simulink model "MASH20_Bader_fixed_point2"  (R2024a)
settings: Solver=ode45  StartTime=0.0  StopTime=1  MaxStep=Ts/10  EnableMultiTasking=on
PreLoadFcn:
  | s0=sprintf('===========================================================================');disp(s0)
  | s1=sprintf('= Created by Bader Almutair bmutairi@kacst.edu.sa                         =');disp(s1)
  | s2=sprintf('= Date 12/11/2014                                                         =');disp(s2)
  | s3=sprintf('= Refer to the PhD thesis Ch4,P.55                                        =');disp(s3)
  | s4=sprintf('===========================================================================');disp(s4)
values from neighbouring files (symbols this model uses):
  AA = AA_design*(mismatch_lower_limit + rand_range*rand)    [simon_test.m]    (also in testPSD_simulink.m)
  acceleration_enable = 1    [simon_test.m]    (also in testPSD_simulink.m)
  b = b_design*(0.8 + (1.2 - 0.8) * rand)    [D2_parameter_mapping.m]    (also in simon_test.m = b_design*(mismatch_lower_limit + rand_range*rand); testPSD_simulink.m = b_design*(mismatch_lower_limit + rand_range*rand))
  clk = i    [GA_multipleruns_TB.m]    (also in GA_multipleruns_TB_c2d.m)
  d0 = d0_design*(mismatch_lower_limit + rand_range*rand)    [simon_test.m]    (also in testPSD_simulink.m)
  electronic_noise_enable = 1    [simon_test.m]    (also in testPSD_simulink.m)
  enoise = 10e-9    (= 1e-08)    [simon_test.m]    (also in testPSD_simulink.m)
  epsilon = 8.854e-12    [population_score_c2d.m]    (also in simon_test.m; testPSD_c2d.m; testPSD_simulink.m)
  Finput = F_resolution*128    (= 260.4140625)    [new_generation_coeff.m]    (also in simon_test.m; testPSD_simulink.m)
  k = k_design*(0.8 + (1.2 - 0.8) * rand)    [D2_parameter_mapping.m]    (also in log2_linear_taylor.m = floor(log2(x)); population_score.m = floor(log2(real(Y3).^2 + imag(Y3).^2)); population_score_c2d.m = floor(log2(Y3)); simon_test.m = k_design*(mismatch_lower_limit + rand_range*rand))
  Kfb = Kfb_design*(0.8 + (1.2 - 0.8) * rand)    [D2_parameter_mapping.m]    (also in simon_test.m = 0.5*epsilon*AA*(Vfeedback^2)/(d0^2); testPSD_simulink.m = 0.5*epsilon*AA*(Vfeedback^2)/(d0^2))
  Kpo = Kpo_design*(0.8 + (1.2 - 0.8) * rand)    [D2_parameter_mapping.m]    (also in simon_test.m = Kpo_design*(mismatch_lower_limit + rand_range*rand); testPSD_simulink.m = Kpo_design*(mismatch_lower_limit + rand_range*rand))
  Lfactor = Vfeedback/d0    [simon_test.m]    (also in testPSD_simulink.m)
  m = m_design*(0.8 + (1.2 - 0.8) * rand)    [D2_parameter_mapping.m]    (also in simon_test.m = m_design*(mismatch_lower_limit + rand_range*rand); testPSD_simulink.m = m_design*(mismatch_lower_limit + rand_range*rand))
  Ts = 1/Fs    (= 7.50007500075e-06)    [new_generation_coeff.m]    (also in simon_test.m; simple_fft_test.m = 1/F; testPSD_c2d.m; testPSD_simulink.m)
  Vfeedback = Vfeedback_design*(mismatch_lower_limit + rand_range*rand)    [simon_test.m]    (also in testPSD_simulink.m)
  x = linspace(min(a4), max(a4), 100)    [D2_parameter_mapping.m]    (also in log2_linear_taylor.m = 1e-10; simon_test.m = 0.9; testPSD_simulink.m = 0.9)
undefined symbols (not defined in the file or in its folder): clk_enable, D2den, reset_x
libraries: hdlmdlgenlib x4, simulink x3, simulink_extras x2, dspsigops x1, vivadosimlib x1
settings Model: Creator=Administrator  LastModifiedBy=Simon
settings SolverCC: AlgebraicLoopSolver=TrustRegion
settings DataIOCC: LimitDataPoints=on  SaveFormat=Array  SignalLoggingSaveFormat=ModelDataLogs  ReturnWorkspaceOutputs=off
settings OptimizationCC: ReuseModelBlockBuffer=off  ExpressionDepthLimit=2147483647  LifeSpan=inf
settings DebuggingCC: UnderspecifiedInitializationDetection=Classic  MergeDetectMultiDrivingBlocksExec=none  SolverPrmCheckMsg=warning  FcnCallInpInsideContextMsg=warning  UnconnectedInputMsg=warning  UnconnectedOutputMsg=warning  UnconnectedLineMsg=warning  StateNameClashWarn=warning  SFUnexpectedBacktrackingDiag=warning  SFNoUnconditionalDefaultTransitionDiag=warning  SFExecutionAtInitializationDiag=none  ArithmeticOperatorsInVariantConditions=warning
settings HardwareCC: ProdBitPerPointer=32  ProdBitPerSizeT=32  ProdBitPerPtrDiffT=32  ProdLargestAtomicFloat=None  ProdIntDivRoundTo=Undefined  ProdEndianess=Unspecified  ProdWordSize=32  ProdHWDeviceType=32-bit Generic
settings ModelReferenceCC: PropagateSignalLabelsOutOfModel=off
settings SFSimCC: SimUseLocalCustomCode=off  CustomCodeUndefinedFunction=UseInterfaceOnly
settings RTWCC: RTWUseLocalCustomCode=off  GPUComputeCapability=3.5
settings CodeAppCC: StateflowObjectComments=on
settings GRTTargetCC: TargetLangStandard=C89/C90 (ANSI)  CombineOutputUpdateFcns=off  GRTInterface=on
settings ConfigComp: CovMetricSettings=dw  CovSaveCumulativeToWorkspaceVar=on  CovSaveSingleToWorkspaceVar=on  CovExternalEMLEnable=off

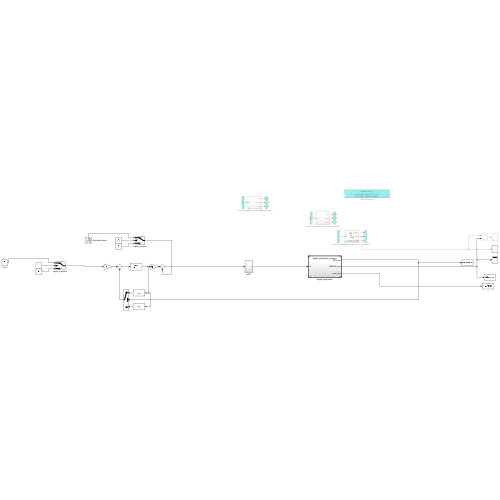
[thumbnail: Simulink's stored preview of the top-level diagram]
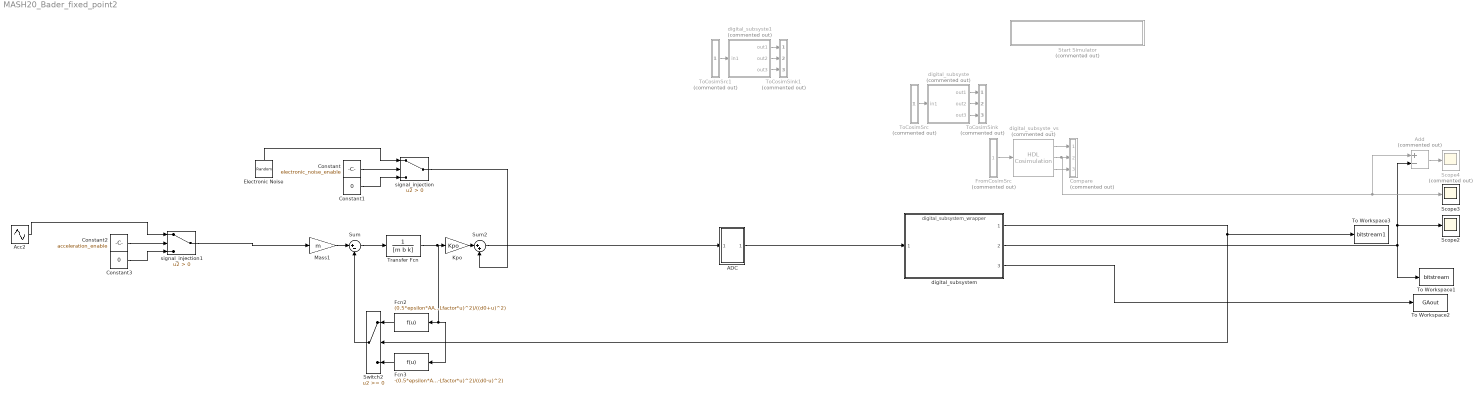
== system MASH20_Bader_fixed_point2 ==
  ADC : Subsystem
  Acc2 : Sin  Amplitude=(Kfb/m)*x  Frequency=Finput*2*pi  SampleTime=0
  Add : Sum  Commented=on  Inputs=+-
  Compare : Subsystem  Commented=on
      mask Display: disp('')
  Constant : Constant  Value=electronic_noise_enable  OutDataTypeStr=boolean  SampleTime=Ts
  Constant1 : Constant  Value=0  OutDataTypeStr=boolean  SampleTime=Ts
  Constant2 : Constant  Value=acceleration_enable  OutDataTypeStr=boolean  SampleTime=Ts
  Constant3 : Constant  Value=0  OutDataTypeStr=boolean  SampleTime=Ts
  Electronic Noise : RandomNumber  Variance=(enoise*sqrt(5/Ts))^2  Seed=432  SampleTime=Ts
  Fcn2 : Fcn  Expr=(0.5*epsilon*AA*(Vfeedback+Lfactor*u)^2)/((d0+u)^2)
  Fcn3 : Fcn  Expr=-(0.5*epsilon*AA*(Vfeedback-Lfactor*u)^2)/((d0-u)^2)
  FromCosimSrc : Subsystem  Commented=on
      mask Display: disp('')
  Kpo : Gain  Gain=Kpo
  Mass1 : Gain  Gain=m
  Scope2 : Scope
  Scope3 : Scope
  Scope4 : Scope  Commented=on
  Start Simulator : Subsystem  Commented=on
      settings: OpenFcn=|
      | cosimDirName = pwd;
      | cd 'hdl_prj_xd\hdlsrc\digital_subsystem_wrapper';
      | [s,r] = system('vivado -mode batch -source gm_digital_subsystem_wrapper_vs.tcl','-echo');
      | cd (cosimDirName);
      | clear cosimDirName;
      | if s
      |    error('Failed to create Vivado HDL design DLL using script gm_digital_subsystem_wrapper_vs.tcl.');
      | end
      mask Display: disp('Double-click to\nregenerate Vivado HDL DLL\nfor design digital_subsyste')
  Sum : Sum  Inputs=|+-
  Sum2 : Sum  Inputs=|++
  Switch2 : Switch  SaturateOnIntegerOverflow=off  InputSameDT=off
  To Workspace1 : ToWorkspace  VariableName=bitstream  SampleTime=Ts
  To Workspace2 : ToWorkspace  VariableName=GAout  SampleTime=Ts
  To Workspace3 : ToWorkspace  VariableName=bitstream1  SampleTime=Ts
  ToCosimSink : Subsystem  Commented=on
      mask Display: disp('')
  ToCosimSink1 : Subsystem  Commented=on
      mask Display: disp('')
  ToCosimSrc : Subsystem  Commented=on
      mask Display: disp('')
  ToCosimSrc1 : Subsystem  Commented=on
      mask Display: disp('')
  Transfer Fcn : TransferFcn  Denominator=[m b k]
  digital_subsyste : Subsystem  Commented=on
  digital_subsyste1 : Subsystem  Commented=on
  digital_subsyste_vs : vivadosimlib/HDL Cosimulation  Commented=on  PortPaths=/digital_subsyste/in1;/digital_subsyste/out1;/digital_subsyste/out2;/digital_subsyste/out3  PortModes=[1 2 2 2 ]  PortTimes=[-1 7.5000750007500073716719922456430680313133052550256252288818359375e-06 7.5000750007500073716719922456430680313133052550256252288818359375e-06 7.5000750007500073716719922456430680313133052550256252288818359375e-06 ]  PortSigns=[-1 1 1 1 ]  PortFracLengths=[0,32,32,32]  PortWordLengths=[-1,64,64,64]  PortHDLWordSizes=[64,64,64,64]  CommLocal=on  CommSharedMemory=on  CommPortNumber=4449  CommShowInfo=on  ClockPaths=clk;clk_enable;reset_x;  ClockModes=[2 4 4]  ClockTimes=[1e-08 3.7e-08 2.7e-08]  TclPreSimCommand="puts \"Running Simulink Cosimulation block.\""  TclPostSimCommand="puts \"done\""  TimingMode=ns  TimingScaleFactor=1333320  idxCellArray={'UNUSED_VAR'}  CosimBypass=Full Simulation  AllowDirectFeedthrough=on  ProductName=EDA Simulator Link VS  RunAutoTimescale=off  HdlClocks=0  PreRunTime=40  PreRunTimeUnit=ns
  digital_subsystem : ModelReference  ModelNameDialog=digital_subsystem_wrapper  SimulationMode=Normal  ModelReferenceVersion=24.17
  signal_injection : Switch  Criteria=u2 > Threshold  SaturateOnIntegerOverflow=off  InputSameDT=off  OutDataTypeStr=Inherit: Same as first input
  signal_injection1 : Switch  Criteria=u2 > Threshold  SaturateOnIntegerOverflow=off  InputSameDT=off  OutDataTypeStr=Inherit: Same as first input
  wires:
  Transfer Fcn/1 -> Fcn3/1, Fcn2/1, Kpo/1
  Sum/1 -> Transfer Fcn/1
  Mass1/1 -> Sum/1
  Fcn2/1 -> Switch2/1
  Fcn3/1 -> Switch2/3
  Switch2/1 -> Sum/2
  Kpo/1 -> Sum2/1
  digital_subsystem/1 -> Switch2/2, To Workspace3/1
  digital_subsystem/2 -> To Workspace1/1, Add/2, Scope2/1
  digital_subsystem/3 -> To Workspace2/1
  digital_subsyste_vs/2 -> Add/1, Scope3/1, Compare/2(in2)
  FromCosimSrc/1(out1) -> digital_subsyste_vs/1
  digital_subsyste_vs/3 -> Compare/3(in3)
  digital_subsyste_vs/1 -> Compare/1(in1)
  Add/1 -> Scope4/1
  Sum2/1 -> ADC/1(In1)
  digital_subsyste/2(out2) -> ToCosimSink/2(in2)
  digital_subsyste/1(out1) -> ToCosimSink/1(in1)
  ToCosimSrc/1(out1) -> digital_subsyste/1(in1)
  digital_subsyste/3(out3) -> ToCosimSink/3(in3)
  ADC/1(Out1) -> digital_subsystem/1
  ToCosimSrc1/1(out1) -> digital_subsyste1/1(in1)
  digital_subsyste1/1(out1) -> ToCosimSink1/1(in1)
  digital_subsyste1/3(out3) -> ToCosimSink1/3(in3)
  digital_subsyste1/2(out2) -> ToCosimSink1/2(in2)
  Constant1/1 -> signal_injection/3
  Electronic Noise/1 -> signal_injection/1
  Constant/1 -> signal_injection/2
  signal_injection/1 -> Sum2/2
  Constant2/1 -> signal_injection1/2
  Acc2/1 -> signal_injection1/1
  Constant3/1 -> signal_injection1/3
  signal_injection1/1 -> Mass1/1

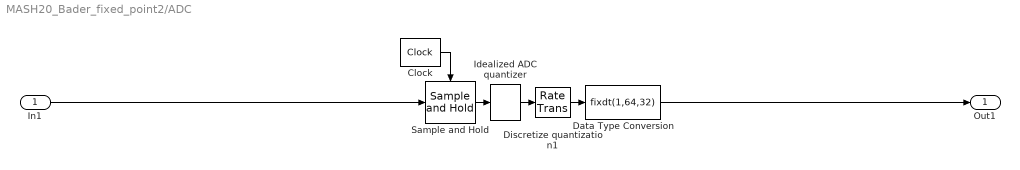
== system MASH20_Bader_fixed_point2/ADC ==
  In1 : Inport
  Clock : simulink_extras/Flip Flops/Clock  period=Ts
  Data Type Conversion : DataTypeConversion  OutDataTypeStr=fixdt(1,64,32)  SaturateOnIntegerOverflow=off  RndMeth=Floor
  Discretize quantization1 : RateTransition  OutPortSampleTime=Ts
  Idealized ADC quantizer : simulink_extras/Additional Discrete/Idealized ADC quantizer  NumberOfConverterBits=12  Vmin=-2.5  Vmax=2.5  OutputDataType=double  OutputNegativeValues=on
  Sample and Hold : dspsigops/Sample and Hold  trig=Rising edge  initCond=0  latchinput=off
  Out1 : Outport
  wires:
  Discretize quantization1/1 -> Data Type Conversion/1
  Idealized ADC quantizer/1 -> Discretize quantization1/1
  Clock/1 -> Sample and Hold/Trigger
  In1/1 -> Sample and Hold/1
  Data Type Conversion/1 -> Out1/1
  Sample and Hold/1 -> Idealized ADC quantizer/1

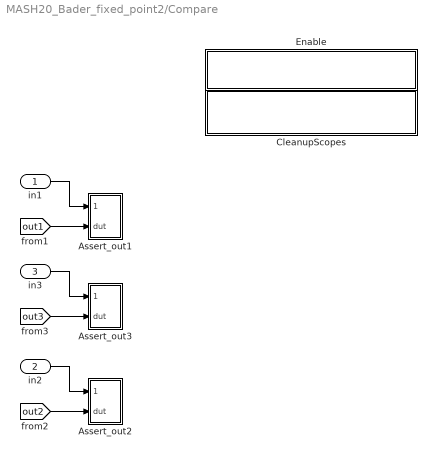
== system MASH20_Bader_fixed_point2/Compare ==
  in1 : Inport
  in2 : Inport  Port=2
  in3 : Inport  Port=3
  Assert_out1 : Subsystem
      settings: LibrarySourceBlock=hdlmdlgenlib/AssertEq
  Assert_out2 : Subsystem
      settings: LibrarySourceBlock=hdlmdlgenlib/AssertEq
  Assert_out3 : Subsystem
      settings: LibrarySourceBlock=hdlmdlgenlib/AssertEq
  CleanupScopes : Subsystem
      settings: OpenFcn=|
      | blkName = gcb; %self block
      | idx = regexp(blkName, '/CleanupScopes$', 'once');
      | blkParent = blkName(1:idx-1);
      | blks=find_system(blkParent, 'LookUnderMasks', 'all','blocktype', 'Scope');
      | for itr = 1:length(blks)
      | 	 hScopeCfg = get_param(blks{itr},'ScopeConfiguration');
      | 	 hScopeCfg.Visible = ~ hScopeCfg.Visible;
      | end
      | drawnow;
      mask Display: fprintf(message('hdlcoder:cosim:vnl_dblclick').getString());
  Enable : Subsystem
      settings: OpenFcn=|
      | blkName = gcb;
      | idx = regexp(blkName, '/Enable$', 'once');
      | blkParent = blkName(1:idx-1);
      | blks=find_system(blkParent, 'LookUnderMasks', 'all','blocktype', 'Assertion');
      | e = get_param(blks{1}, 'Enabled');
      | if strcmp(e, 'on'), f= 'off';, else, f = 'on';, end
      | for ii=1:length(blks), set_param(blks{ii}, 'Enabled', f);, end
      | set_param(gcb, 'MaskDisplay',['fprintf(message(''hdlcoder:cosim:vnl_dblclick_assertions'',','''',upper(e),'''',').getString())']);
      mask Display: fprintf(message('hdlcoder:cosim:vnl_dblclick_assertions','OFF').getString());
  wires:
  [out3] -> Assert_out3/2(dut)
  in3/1 -> Assert_out3/1(cosim)
  in1/1 -> Assert_out1/1(cosim)
  in2/1 -> Assert_out2/1(cosim)
  [out1] -> Assert_out1/2(dut)
  [out2] -> Assert_out2/2(dut)

== system MASH20_Bader_fixed_point2/FromCosimSrc ==
  out1 : Outport
  wires:
  [in1] -> out1/1

== system MASH20_Bader_fixed_point2/Start Simulator ==

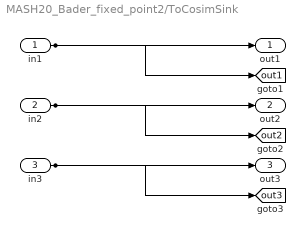
== system MASH20_Bader_fixed_point2/ToCosimSink ==
  in1 : Inport
  in2 : Inport  Port=2
  in3 : Inport  Port=3
  out1 : Outport
  out2 : Outport  Port=2
  out3 : Outport  Port=3
  tag scope: out1=global, out2=global, out3=global
  wires:
  in1/1 -> out1/1, [out1]
  in2/1 -> out2/1, [out2]
  in3/1 -> out3/1, [out3]

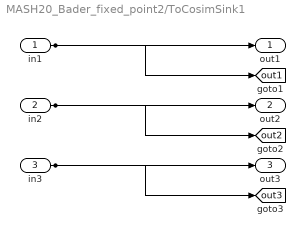
== system MASH20_Bader_fixed_point2/ToCosimSink1 ==
  in1 : Inport
  in2 : Inport  Port=2
  in3 : Inport  Port=3
  out1 : Outport
  out2 : Outport  Port=2
  out3 : Outport  Port=3
  tag scope: out1=global, out2=global, out3=global
  wires:
  in1/1 -> out1/1, [out1]
  in2/1 -> out2/1, [out2]
  in3/1 -> out3/1, [out3]

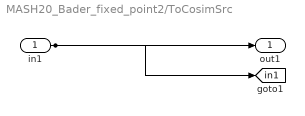
== system MASH20_Bader_fixed_point2/ToCosimSrc ==
  in1 : Inport
  out1 : Outport
  tag scope: in1=global
  wires:
  in1/1 -> out1/1, [in1]

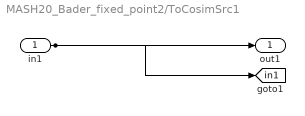
== system MASH20_Bader_fixed_point2/ToCosimSrc1 ==
  in1 : Inport
  out1 : Outport
  tag scope: in1=global
  wires:
  in1/1 -> out1/1, [in1]

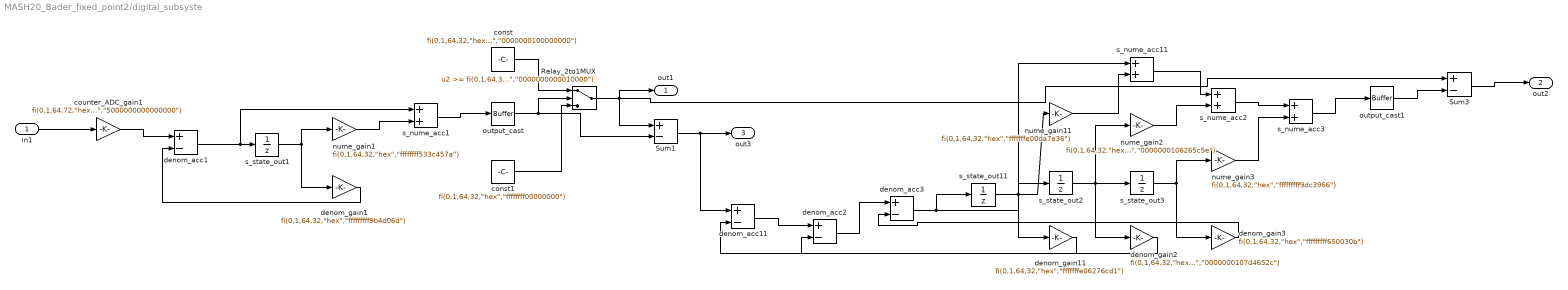
== system MASH20_Bader_fixed_point2/digital_subsyste ==
  in1 : Inport  OutDataTypeStr=fixdt(1, 64, 32)  PortDimensions=1  SampleTime=7.50007500075001e-06
  Relay_2to1MUX : Switch  Threshold="fi(0,1,64,32,\"hex\",\"0000000000010000\")"  OutDataTypeStr=fixdt(1, 64, 32)  SampleTime=7.50007500075001e-06  SaturateOnIntegerOverflow=off  InputSameDT=off
  Sum1 : Sum  Inputs=+-  OutDataTypeStr=fixdt(1, 64, 32)  AccumDataTypeStr=fixdt(1, 64, 32)  SampleTime=7.50007500075001e-06
  Sum3 : Sum  Inputs=+-  OutDataTypeStr=fixdt(1, 64, 32)  AccumDataTypeStr=fixdt(1, 64, 32)  SampleTime=7.50007500075001e-06
  const : Constant  Value="fi(0,1,64,32,\"hex\",\"0000000100000000\")"  OutDataTypeStr=fixdt(1, 64, 32)  SampleTime=7.50007500075001e-06
  const1 : Constant  Value="fi(0,1,64,32,\"hex\",\"ffffffff00000000\")"  OutDataTypeStr=fixdt(1, 64, 32)  SampleTime=7.50007500075001e-06
  counter_ADC_gain1 : Gain  Gain="fi(0,1,64,72,\"hex\",\"5000000000000000\")"  ParamDataTypeStr=fixdt(1, 64, 72)  OutDataTypeStr=fixdt(1, 64, 32)  SampleTime=7.50007500075001e-06
  denom_acc{1..3,11} (4 alike) : Sum  Inputs=+-  OutDataTypeStr=fixdt(1, 64, 32)  AccumDataTypeStr=fixdt(1, 64, 32)  SampleTime=7.50007500075001e-06
  denom_gain1 : Gain  Gain="fi(0,1,64,32,\"hex\",\"fffffffff9b4d06d\")"  ParamDataTypeStr=fixdt(1, 64, 32)  OutDataTypeStr=fixdt(1, 64, 32)  SampleTime=7.50007500075001e-06
  denom_gain11 : Gain  Gain="fi(0,1,64,32,\"hex\",\"fffffffe06276cd1\")"  ParamDataTypeStr=fixdt(1, 64, 32)  OutDataTypeStr=fixdt(1, 64, 32)  SampleTime=7.50007500075001e-06
  denom_gain2 : Gain  Gain="fi(0,1,64,32,\"hex\",\"0000000107d4652c\")"  ParamDataTypeStr=fixdt(1, 64, 32)  OutDataTypeStr=fixdt(1, 64, 32)  SampleTime=7.50007500075001e-06
  denom_gain3 : Gain  Gain="fi(0,1,64,32,\"hex\",\"fffffffff650030b\")"  ParamDataTypeStr=fixdt(1, 64, 32)  OutDataTypeStr=fixdt(1, 64, 32)  SampleTime=7.50007500075001e-06
  nume_gain1 : Gain  Gain="fi(0,1,64,32,\"hex\",\"ffffffff533c457a\")"  ParamDataTypeStr=fixdt(1, 64, 32)  OutDataTypeStr=fixdt(1, 64, 32)  SampleTime=7.50007500075001e-06
  nume_gain11 : Gain  Gain="fi(0,1,64,32,\"hex\",\"fffffffe00da7e36\")"  ParamDataTypeStr=fixdt(1, 64, 32)  OutDataTypeStr=fixdt(1, 64, 32)  SampleTime=7.50007500075001e-06
  nume_gain2 : Gain  Gain="fi(0,1,64,32,\"hex\",\"0000000106265c5e\")"  ParamDataTypeStr=fixdt(1, 64, 32)  OutDataTypeStr=fixdt(1, 64, 32)  SampleTime=7.50007500075001e-06
  nume_gain3 : Gain  Gain="fi(0,1,64,32,\"hex\",\"fffffffff9dc3966\")"  ParamDataTypeStr=fixdt(1, 64, 32)  OutDataTypeStr=fixdt(1, 64, 32)  SampleTime=7.50007500075001e-06
  output_cast : hdlmdlgenlib/Buffer
  output_cast1 : hdlmdlgenlib/Buffer
  s_nume_acc{1..3,11} (4 alike) : Sum  OutDataTypeStr=fixdt(1, 64, 32)  SampleTime=7.50007500075001e-06
  s_state_out{1..3,11} (4 alike) : UnitDelay  InitialCondition="fi(0,1,64,32,\"hex\",\"0000000000000000\")"  SampleTime=7.50007500075001e-06
  out1 : Outport  SampleTime=7.50007500075001e-06
  out2 : Outport  Port=2  SampleTime=7.50007500075001e-06
  out3 : Outport  Port=3  SampleTime=7.50007500075001e-06
  wires:
  const1/1 -> Relay_2to1MUX/3
  const/1 -> Relay_2to1MUX/1
  output_cast1/1 -> Sum3/2
  s_nume_acc3/1 -> output_cast1/1
  s_nume_acc2/1 -> s_nume_acc3/1
  s_nume_acc11/1 -> s_nume_acc2/1
  nume_gain3/1 -> s_nume_acc3/2
  nume_gain2/1 -> s_nume_acc2/2
  nume_gain11/1 -> s_nume_acc11/2
  denom_gain3/1 -> denom_acc3/2
  denom_gain2/1 -> denom_acc2/2
  denom_gain11/1 -> denom_acc11/2
  s_state_out3/1 -> denom_gain3/1, nume_gain3/1
  s_state_out2/1 -> s_state_out3/1, denom_gain2/1, nume_gain2/1
  s_state_out11/1 -> s_state_out2/1, denom_gain11/1, nume_gain11/1
  denom_acc3/1 -> s_nume_acc11/1, s_state_out11/1
  denom_acc2/1 -> denom_acc3/1
  denom_acc11/1 -> denom_acc2/1
  output_cast/1 -> Relay_2to1MUX/2, Sum1/2
  s_nume_acc1/1 -> output_cast/1
  nume_gain1/1 -> s_nume_acc1/2
  denom_gain1/1 -> denom_acc1/2
  s_state_out1/1 -> denom_gain1/1, nume_gain1/1
  denom_acc1/1 -> s_nume_acc1/1, s_state_out1/1
  counter_ADC_gain1/1 -> denom_acc1/1
  Sum3/1 -> out2/1
  Sum1/1 -> denom_acc11/1, out3/1
  Relay_2to1MUX/1 -> out1/1, Sum1/1, Sum3/1
  in1/1 -> counter_ADC_gain1/1

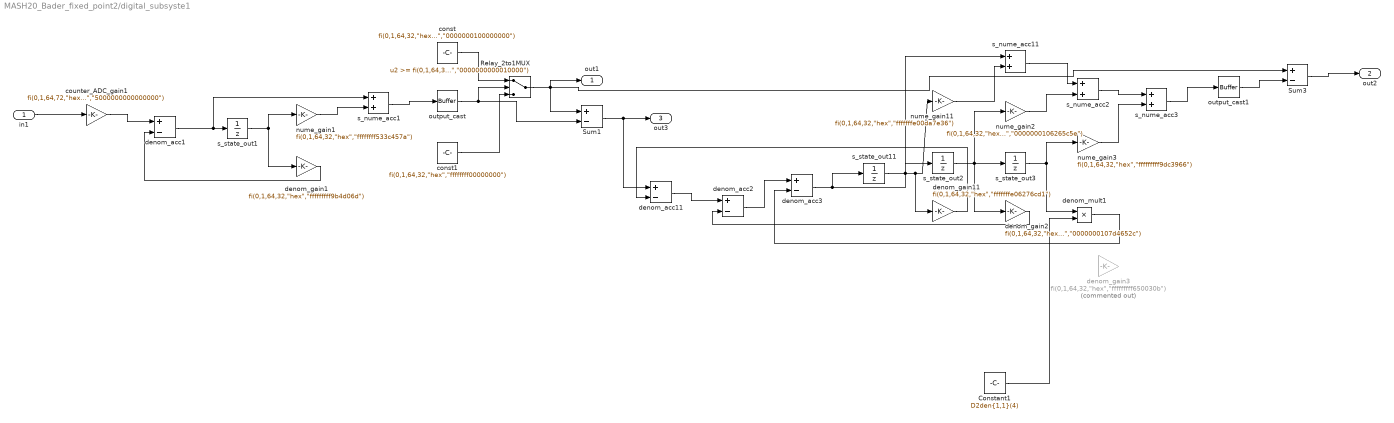
== system MASH20_Bader_fixed_point2/digital_subsyste1 ==
  in1 : Inport  OutDataTypeStr=fixdt(1, 64, 32)  PortDimensions=1  SampleTime=7.50007500075001e-06
  Constant1 : Constant  Value=D2den{1,1}(4)  OutDataTypeStr=fixdt(1,64,32)  SampleTime=Ts
  Relay_2to1MUX : Switch  Threshold="fi(0,1,64,32,\"hex\",\"0000000000010000\")"  OutDataTypeStr=fixdt(1, 64, 32)  SampleTime=7.50007500075001e-06  SaturateOnIntegerOverflow=off  InputSameDT=off
  Sum1 : Sum  Inputs=+-  OutDataTypeStr=fixdt(1, 64, 32)  AccumDataTypeStr=fixdt(1, 64, 32)  SampleTime=7.50007500075001e-06
  Sum3 : Sum  Inputs=+-  OutDataTypeStr=fixdt(1, 64, 32)  AccumDataTypeStr=fixdt(1, 64, 32)  SampleTime=7.50007500075001e-06
  const : Constant  Value="fi(0,1,64,32,\"hex\",\"0000000100000000\")"  OutDataTypeStr=fixdt(1, 64, 32)  SampleTime=7.50007500075001e-06
  const1 : Constant  Value="fi(0,1,64,32,\"hex\",\"ffffffff00000000\")"  OutDataTypeStr=fixdt(1, 64, 32)  SampleTime=7.50007500075001e-06
  counter_ADC_gain1 : Gain  Gain="fi(0,1,64,72,\"hex\",\"5000000000000000\")"  ParamDataTypeStr=fixdt(1, 64, 72)  OutDataTypeStr=fixdt(1, 64, 32)  SampleTime=7.50007500075001e-06
  denom_acc{1..3,11} (4 alike) : Sum  Inputs=+-  OutDataTypeStr=fixdt(1, 64, 32)  AccumDataTypeStr=fixdt(1, 64, 32)  SampleTime=7.50007500075001e-06
  denom_gain1 : Gain  Gain="fi(0,1,64,32,\"hex\",\"fffffffff9b4d06d\")"  ParamDataTypeStr=fixdt(1, 64, 32)  OutDataTypeStr=fixdt(1, 64, 32)  SampleTime=7.50007500075001e-06
  denom_gain11 : Gain  Gain="fi(0,1,64,32,\"hex\",\"fffffffe06276cd1\")"  ParamDataTypeStr=fixdt(1, 64, 32)  OutDataTypeStr=fixdt(1, 64, 32)  SampleTime=7.50007500075001e-06
  denom_gain2 : Gain  Gain="fi(0,1,64,32,\"hex\",\"0000000107d4652c\")"  ParamDataTypeStr=fixdt(1, 64, 32)  OutDataTypeStr=fixdt(1, 64, 32)  SampleTime=7.50007500075001e-06
  denom_gain3 : Gain  Commented=on  Gain="fi(0,1,64,32,\"hex\",\"fffffffff650030b\")"  ParamDataTypeStr=fixdt(1, 64, 32)  OutDataTypeStr=fixdt(1, 64, 32)  SampleTime=7.50007500075001e-06
  denom_mult1 : Product  OutDataTypeStr=fixdt(1,64,32)
  nume_gain1 : Gain  Gain="fi(0,1,64,32,\"hex\",\"ffffffff533c457a\")"  ParamDataTypeStr=fixdt(1, 64, 32)  OutDataTypeStr=fixdt(1, 64, 32)  SampleTime=7.50007500075001e-06
  nume_gain11 : Gain  Gain="fi(0,1,64,32,\"hex\",\"fffffffe00da7e36\")"  ParamDataTypeStr=fixdt(1, 64, 32)  OutDataTypeStr=fixdt(1, 64, 32)  SampleTime=7.50007500075001e-06
  nume_gain2 : Gain  Gain="fi(0,1,64,32,\"hex\",\"0000000106265c5e\")"  ParamDataTypeStr=fixdt(1, 64, 32)  OutDataTypeStr=fixdt(1, 64, 32)  SampleTime=7.50007500075001e-06
  nume_gain3 : Gain  Gain="fi(0,1,64,32,\"hex\",\"fffffffff9dc3966\")"  ParamDataTypeStr=fixdt(1, 64, 32)  OutDataTypeStr=fixdt(1, 64, 32)  SampleTime=7.50007500075001e-06
  output_cast : hdlmdlgenlib/Buffer
  output_cast1 : hdlmdlgenlib/Buffer
  s_nume_acc{1..3,11} (4 alike) : Sum  OutDataTypeStr=fixdt(1, 64, 32)  SampleTime=7.50007500075001e-06
  s_state_out{1..3,11} (4 alike) : UnitDelay  InitialCondition="fi(0,1,64,32,\"hex\",\"0000000000000000\")"  SampleTime=7.50007500075001e-06
  out1 : Outport  SampleTime=7.50007500075001e-06
  out2 : Outport  Port=2  SampleTime=7.50007500075001e-06
  out3 : Outport  Port=3  SampleTime=7.50007500075001e-06
  wires:
  const1/1 -> Relay_2to1MUX/3
  const/1 -> Relay_2to1MUX/1
  output_cast1/1 -> Sum3/2
  s_nume_acc3/1 -> output_cast1/1
  s_nume_acc2/1 -> s_nume_acc3/1
  s_nume_acc11/1 -> s_nume_acc2/1
  nume_gain3/1 -> s_nume_acc3/2
  nume_gain2/1 -> s_nume_acc2/2
  nume_gain11/1 -> s_nume_acc11/2
  denom_mult1/1 -> denom_acc3/2
  denom_gain2/1 -> denom_acc2/2
  denom_gain11/1 -> denom_acc11/2
  s_state_out3/1 -> denom_mult1/1, nume_gain3/1
  s_state_out2/1 -> s_state_out3/1, denom_gain2/1, nume_gain2/1
  s_state_out11/1 -> denom_gain11/1, nume_gain11/1, s_state_out2/1
  denom_acc3/1 -> s_nume_acc11/1, s_state_out11/1
  denom_acc2/1 -> denom_acc3/1
  denom_acc11/1 -> denom_acc2/1
  output_cast/1 -> Relay_2to1MUX/2, Sum1/2
  s_nume_acc1/1 -> output_cast/1
  nume_gain1/1 -> s_nume_acc1/2
  denom_gain1/1 -> denom_acc1/2
  s_state_out1/1 -> denom_gain1/1, nume_gain1/1
  denom_acc1/1 -> s_nume_acc1/1, s_state_out1/1
  counter_ADC_gain1/1 -> denom_acc1/1
  Sum3/1 -> out2/1
  Sum1/1 -> denom_acc11/1, out3/1
  Relay_2to1MUX/1 -> out1/1, Sum1/1, Sum3/1
  in1/1 -> counter_ADC_gain1/1
  Constant1/1 -> denom_mult1/2

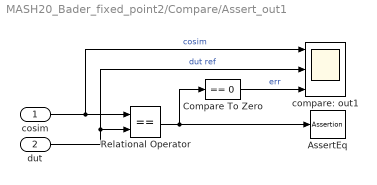
== system MASH20_Bader_fixed_point2/Compare/Assert_out1 ==
  cosim : Inport
  dut : Inport  Port=2
  AssertEq : Assertion  StopWhenAssertionFail=off
  Compare To Zero : simulink/Logic and Bit Operations/Compare To Zero  relop===  OutDataTypeStr=boolean
  Relational Operator : RelationalOperator  Operator===  OutDataTypeStr=boolean  InputSameDT=off
  compare: out1 : Scope  NumInputPorts=3
  wires:
  Compare To Zero/1 -> compare: out1/3  "err"
  Relational Operator/1 -> Compare To Zero/1, AssertEq/1
  cosim/1 -> compare: out1/1, Relational Operator/1  "cosim"
  dut/1 -> compare: out1/2, Relational Operator/2  "dut ref"

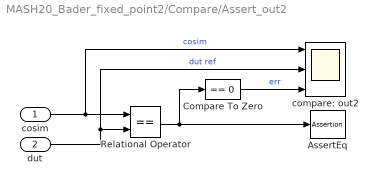
== system MASH20_Bader_fixed_point2/Compare/Assert_out2 ==
  cosim : Inport
  dut : Inport  Port=2
  AssertEq : Assertion  StopWhenAssertionFail=off
  Compare To Zero : simulink/Logic and Bit Operations/Compare To Zero  relop===  OutDataTypeStr=boolean
  Relational Operator : RelationalOperator  Operator===  OutDataTypeStr=boolean  InputSameDT=off
  compare: out2 : Scope  NumInputPorts=3
  wires:
  Compare To Zero/1 -> compare: out2/3  "err"
  Relational Operator/1 -> Compare To Zero/1, AssertEq/1
  cosim/1 -> compare: out2/1, Relational Operator/1  "cosim"
  dut/1 -> compare: out2/2, Relational Operator/2  "dut ref"

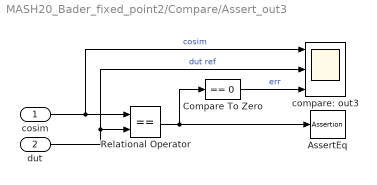
== system MASH20_Bader_fixed_point2/Compare/Assert_out3 ==
  cosim : Inport
  dut : Inport  Port=2
  AssertEq : Assertion  StopWhenAssertionFail=off
  Compare To Zero : simulink/Logic and Bit Operations/Compare To Zero  relop===  OutDataTypeStr=boolean
  Relational Operator : RelationalOperator  Operator===  OutDataTypeStr=boolean  InputSameDT=off
  compare: out3 : Scope  NumInputPorts=3
  wires:
  Compare To Zero/1 -> compare: out3/3  "err"
  Relational Operator/1 -> Compare To Zero/1, AssertEq/1
  cosim/1 -> compare: out3/1, Relational Operator/1  "cosim"
  dut/1 -> compare: out3/2, Relational Operator/2  "dut ref"

== system MASH20_Bader_fixed_point2/Compare/CleanupScopes ==

== system MASH20_Bader_fixed_point2/Compare/Enable ==
